simulink model "hpt_1to1_topology"  (R2025a)
settings: Solver=ode23tb  StartTime=0.0  StopTime=0.2  RelTol=1e-3
libraries: spsLinearTransformerLib x9, spsGroundLib x4, spsThreePhaseVIMeasurementLib x3, spsSeriesRLCBranchLib x2, spsThreePhaseSeriesRLCBranchLib x2, spsUniversalBridgeLib x2, spsIGBTLib x1, spsThreePhaseSourceLib x1, spsThreePhaseSeriesRLCLoadLib x1, spsVoltageMeasurementLib x1, spspowerguiLib x1
settings Model: Creator=m1391  LastModifiedBy=m1391

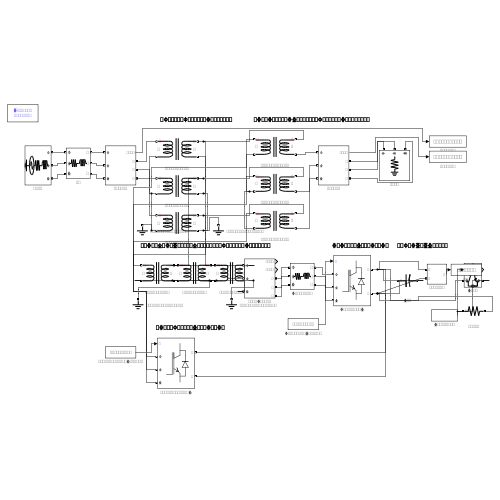
[thumbnail: Simulink's stored preview of the top-level diagram]
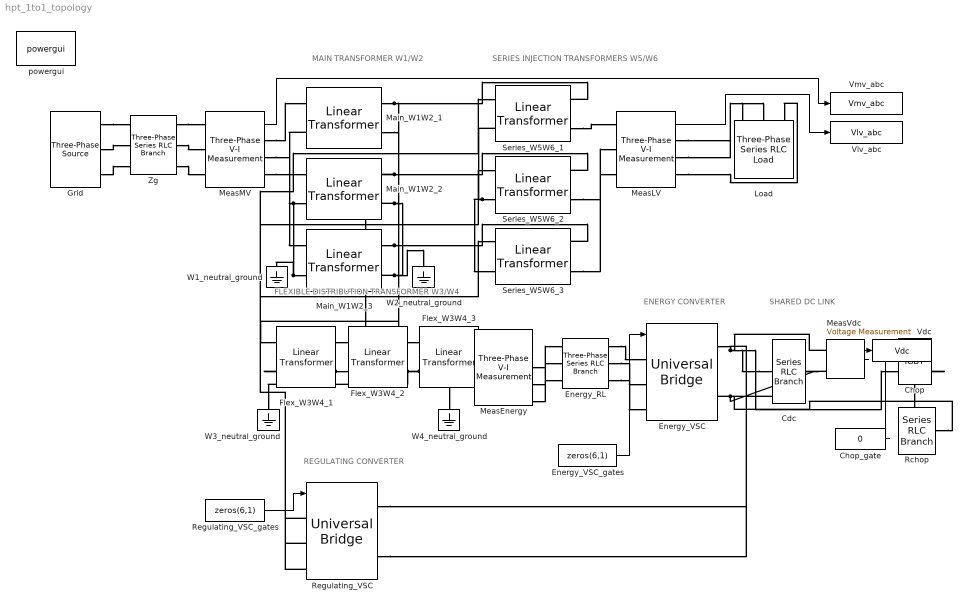
== system hpt_1to1_topology ==
  note: MAIN TRANSFORMER W1/W2
  note: FLEXIBLE DISTRIBUTION TRANSFORMER W3/W4
  note: SERIES INJECTION TRANSFORMERS W5/W6
  note: ENERGY CONVERTER
  note: REGULATING CONVERTER
  note: SHARED DC LINK
  Cdc : spsSeriesRLCBranchLib/Series RLC Branch  LConnTagsString=__new0  RConnTagsString=__new0  BranchType=C  Resistance=1  Inductance=1e-3  SetiL0=off  InitialCurrent=0  Capacitance=0.0022  Setx0=on  InitialVoltage=800  Measurements=None
  Chop : spsIGBTLib/IGBT  Ron=0.001  Lon=0  Vf=1  Tf=1e-6  Tt=2e-6  IC=0  Rs=1e5  Cs=inf  Measurements=on
  Chop_gate : Constant  Value=0
  Energy_RL : spsThreePhaseSeriesRLCBranchLib/Three-Phase Series RLC Branch  LConnTagsString=A|B|C  RConnTagsString=A|B|C  BranchType=RL  Resistance=0.05  Inductance=0.003  Capacitance=1e-6  Measurements=None
  Energy_VSC : spsUniversalBridgeLib/Universal Bridge  Arms=3  SnubberResistance=1e5  SnubberCapacitance=inf  Device=IGBT / Diodes  Ron=1e-3  Lon=0  ForwardVoltages="[  0  0  ]"  ForwardVoltage=0  GTOparameters=[ 10e-6 , 20e-6 ]  IGBTparameters=[ 1e-6 , 2e-6 ]  Measurements=None  Measurements_2=None  converterType=Rectifier
  Energy_VSC_gates : Constant  Value=zeros(6,1)
  Flex_W3W4_1 : spsLinearTransformerLib/Linear Transformer  UNITS=pu  NominalPower=[40000,50]  winding1=[230.9401,0.005,0.02]  winding2=[230.9401,0.005,0.02]  ThreeWindings=off  winding3=[ 315e3 0.002 0.08 ]  RmLm=[ 500 500 ]  Measurements=None  DataType=off
  Flex_W3W4_2 : spsLinearTransformerLib/Linear Transformer  UNITS=pu  NominalPower=[40000,50]  winding1=[230.9401,0.005,0.02]  winding2=[230.9401,0.005,0.02]  ThreeWindings=off  winding3=[ 315e3 0.002 0.08 ]  RmLm=[ 500 500 ]  Measurements=None  DataType=off
  Flex_W3W4_3 : spsLinearTransformerLib/Linear Transformer  UNITS=pu  NominalPower=[40000,50]  winding1=[230.9401,0.005,0.02]  winding2=[230.9401,0.005,0.02]  ThreeWindings=off  winding3=[ 315e3 0.002 0.08 ]  RmLm=[ 500 500 ]  Measurements=None  DataType=off
  Grid : spsThreePhaseSourceLib/Three-Phase Source  InternalConnection=Yg  VoltagePhases=off  Voltage=10000  PhaseAngle=0  Voltage_phases=[25e3 25e3 25e3]/sqrt(3)  PhaseAngles_phases=[0 -120 +120]  Frequency=50  NonIdealSource=on  SpecifyImpedance=off  Resistance=1e-3  Inductance=1e-5  ShortCircuitLevel=100e6  BaseVoltage=25e3  XRratio=7  BusType=swing  Pref=10e3  Qref=0  Prefabc=[10e3, 10e3, 10e3]  Qrefabc=[0, 0, 0]  Qmin=-inf  Qmax=inf
  Load : spsThreePhaseSeriesRLCLoadLib/Three-Phase Series RLC Load  LConnTagsString=A|B|C  Configuration=Y (grounded)  NominalVoltage=400  Vabc=[1e3 1e3 1e3]  Vabcp=[1e3 1e3 1e3]  NominalFrequency=50  UnbalancedPower=off  ActivePower=400000  InductivePower=0  CapacitivePower=0  Pabc=[10e3 9e3 11e3]  QLabc=[100 90 110]  QCabc=[100 90 110]  Pabcp=[10e3 9e3 11e3]  QLabcp=[100 90 110]  QCabcp=[100 90 110]  Measurements=None  LoadType=constant Z
  Main_W1W2_1 : spsLinearTransformerLib/Linear Transformer  UNITS=pu  NominalPower=[133333.3333,50]  winding1=[5773.5027,0.005,0.025]  winding2=[230.9401,0.005,0.025]  ThreeWindings=off  winding3=[ 315e3 0.002 0.08 ]  RmLm=[ 500 500 ]  Measurements=None  DataType=off
  Main_W1W2_2 : spsLinearTransformerLib/Linear Transformer  UNITS=pu  NominalPower=[133333.3333,50]  winding1=[5773.5027,0.005,0.025]  winding2=[230.9401,0.005,0.025]  ThreeWindings=off  winding3=[ 315e3 0.002 0.08 ]  RmLm=[ 500 500 ]  Measurements=None  DataType=off
  Main_W1W2_3 : spsLinearTransformerLib/Linear Transformer  UNITS=pu  NominalPower=[133333.3333,50]  winding1=[5773.5027,0.005,0.025]  winding2=[230.9401,0.005,0.025]  ThreeWindings=off  winding3=[ 315e3 0.002 0.08 ]  RmLm=[ 500 500 ]  Measurements=None  DataType=off
  MeasEnergy : spsThreePhaseVIMeasurementLib/Three-Phase V-I Measurement  VoltageMeasurement=phase-to-ground  SetLabelV=off  LabelV=Vabc  Vpu=off  VpuLL=off  CurrentMeasurement=yes  SetLabelI=off  LabelI=Iabc  Ipu=off  Pbase=100e6  Vbase=500e3  OutputType=Complex  PhasorSimulation=off  PSBequivalent=0
  MeasLV : spsThreePhaseVIMeasurementLib/Three-Phase V-I Measurement  VoltageMeasurement=phase-to-ground  SetLabelV=off  LabelV=Vabc  Vpu=off  VpuLL=off  CurrentMeasurement=no  SetLabelI=off  LabelI=Iabc  Ipu=off  Pbase=100e6  Vbase=500e3  OutputType=Complex  PhasorSimulation=off  PSBequivalent=0
  MeasMV : spsThreePhaseVIMeasurementLib/Three-Phase V-I Measurement  VoltageMeasurement=phase-to-ground  SetLabelV=off  LabelV=Vabc  Vpu=off  VpuLL=off  CurrentMeasurement=no  SetLabelI=off  LabelI=Iabc  Ipu=off  Pbase=100e6  Vbase=500e3  OutputType=Complex  PhasorSimulation=off  PSBequivalent=0
  MeasVdc : spsVoltageMeasurementLib/Voltage Measurement  PhasorSimulation=off  OutputType=Complex  PSBequivalent=0
  Rchop : spsSeriesRLCBranchLib/Series RLC Branch  LConnTagsString=__new0  RConnTagsString=__new0  BranchType=R  Resistance=5.3333  Inductance=1e-3  SetiL0=off  InitialCurrent=0  Capacitance=1e-6  Setx0=off  InitialVoltage=0  Measurements=None
  Regulating_VSC : spsUniversalBridgeLib/Universal Bridge  Arms=3  SnubberResistance=1e5  SnubberCapacitance=inf  Device=IGBT / Diodes  Ron=1e-3  Lon=0  ForwardVoltages="[  0  0  ]"  ForwardVoltage=0  GTOparameters=[ 10e-6 , 20e-6 ]  IGBTparameters=[ 1e-6 , 2e-6 ]  Measurements=None  Measurements_2=None  converterType=Rectifier
  Regulating_VSC_gates : Constant  Value=zeros(6,1)
  Series_W5W6_1 : spsLinearTransformerLib/Linear Transformer  UNITS=pu  NominalPower=[30000,50]  winding1=[400,0.002,0.03]  winding2=[46.2,0.002,0.03]  ThreeWindings=off  winding3=[ 315e3 0.002 0.08 ]  RmLm=[ 500 500 ]  Measurements=None  DataType=off
  Series_W5W6_2 : spsLinearTransformerLib/Linear Transformer  UNITS=pu  NominalPower=[30000,50]  winding1=[400,0.002,0.03]  winding2=[46.2,0.002,0.03]  ThreeWindings=off  winding3=[ 315e3 0.002 0.08 ]  RmLm=[ 500 500 ]  Measurements=None  DataType=off
  Series_W5W6_3 : spsLinearTransformerLib/Linear Transformer  UNITS=pu  NominalPower=[30000,50]  winding1=[400,0.002,0.03]  winding2=[46.2,0.002,0.03]  ThreeWindings=off  winding3=[ 315e3 0.002 0.08 ]  RmLm=[ 500 500 ]  Measurements=None  DataType=off
  Vdc : ToWorkspace  VariableName=Vdc  SampleTime=2e-05
  Vlv_abc : ToWorkspace  VariableName=Vlv_abc  SampleTime=2e-05
  Vmv_abc : ToWorkspace  VariableName=Vmv_abc  SampleTime=2e-05
  W1_neutral_ground : spsGroundLib/Ground  LConnTagsString=a
  W2_neutral_ground : spsGroundLib/Ground  LConnTagsString=a
  W3_neutral_ground : spsGroundLib/Ground  LConnTagsString=a
  W4_neutral_ground : spsGroundLib/Ground  LConnTagsString=a
  Zg : spsThreePhaseSeriesRLCBranchLib/Three-Phase Series RLC Branch  LConnTagsString=A|B|C  RConnTagsString=A|B|C  BranchType=RL  Resistance=11.7851  Inductance=0.26259  Capacitance=1e-6  Measurements=None
  powergui : spspowerguiLib/powergui  Priority=1  SimulationMode=Discrete  SampleTime=2e-05  frequency=60  Iterations=50  frequencyindice=60  Pbase=100e6  ErrMax=1e-4  UnitsV=kV  UnitsW=MW  buscounter=0  FunctionMessages=off  echomessages=off  EnableUseOfTLC=off  CurrentSourceSwitches=off  DisableSnubberDevices=off  DisableRonSwitches=off  DisableVfSwitches=off  DisplayEquations=off  AutomaticDiscreteSolvers=off  SolverType=Tustin/Backward Euler (TBE)  Interpol=off  ExternalGateDelay=off  methode=off  Ts=100  x0status=blocks  SPID=on  SwTol=0  HookPort=off  NonlinearTolerance=1e-4  nMaxIteration=100  ContinueOnMaxIteration=off  RestoreLinks=warning  ResistiveCurrentMeasurement=off  Frange=[0:2:500]  Ylog=off  Xlog=on  ShowGrid=off  save=off  variable=ZData  structure=0  ZoomFFT=off  StartTime=0.0  cycles=1  DisplayStyle=1  fundamental=60  FreqAxis=off  MaxFrequency=1000  frequencyindicesteady=1  RmsSteady=1  display=off
  wires:
  Energy_VSC_gates/1 -> Energy_VSC/1
  Regulating_VSC_gates/1 -> Regulating_VSC/1
  Chop_gate/1 -> Chop/1
  MeasMV/1 -> Vmv_abc/1
  MeasLV/1 -> Vlv_abc/1
  MeasVdc/1 -> Vdc/1
  connections:
  Grid/RConn1 -- Zg/LConn1
  Zg/RConn1 -- MeasMV/LConn1
  MeasMV/RConn1 -- Main_W1W2_1/LConn1
  Series_W5W6_1/RConn1 -- Main_W1W2_1/RConn1 -- Flex_W3W4_1/LConn1
  Series_W5W6_1/RConn2 -- MeasLV/LConn1
  MeasLV/RConn1 -- Load/LConn1
  Flex_W3W4_1/RConn1 -- MeasEnergy/LConn1
  MeasEnergy/RConn1 -- Energy_RL/LConn1
  Energy_RL/RConn1 -- Energy_VSC/LConn1
  Regulating_VSC/LConn1 -- Series_W5W6_1/LConn1
  Grid/RConn2 -- Zg/LConn2
  Zg/RConn2 -- MeasMV/LConn2
  MeasMV/RConn2 -- Main_W1W2_2/LConn1
  Series_W5W6_2/RConn1 -- Main_W1W2_2/RConn1 -- Flex_W3W4_2/LConn1
  Series_W5W6_2/RConn2 -- MeasLV/LConn2
  MeasLV/RConn2 -- Load/LConn2
  Flex_W3W4_2/RConn1 -- MeasEnergy/LConn2
  MeasEnergy/RConn2 -- Energy_RL/LConn2
  Energy_RL/RConn2 -- Energy_VSC/LConn2
  Regulating_VSC/LConn2 -- Series_W5W6_2/LConn1
  Grid/RConn3 -- Zg/LConn3
  Zg/RConn3 -- MeasMV/LConn3
  MeasMV/RConn3 -- Main_W1W2_3/LConn1
  Series_W5W6_3/RConn1 -- Main_W1W2_3/RConn1 -- Flex_W3W4_3/LConn1
  Series_W5W6_3/RConn2 -- MeasLV/LConn3
  MeasLV/RConn3 -- Load/LConn3
  Flex_W3W4_3/RConn1 -- MeasEnergy/LConn3
  MeasEnergy/RConn3 -- Energy_RL/LConn3
  Energy_RL/RConn3 -- Energy_VSC/LConn3
  Regulating_VSC/LConn3 -- Series_W5W6_3/LConn1
  Main_W1W2_2/LConn2 -- Main_W1W2_1/LConn2 -- Main_W1W2_3/LConn2 -- W1_neutral_ground/LConn1
  Main_W1W2_2/RConn2 -- Main_W1W2_1/RConn2 -- Main_W1W2_3/RConn2 -- W2_neutral_ground/LConn1
  Flex_W3W4_2/LConn2 -- Flex_W3W4_1/LConn2 -- Flex_W3W4_3/LConn2 -- W3_neutral_ground/LConn1
  Flex_W3W4_2/RConn2 -- Flex_W3W4_1/RConn2 -- Flex_W3W4_3/RConn2 -- W4_neutral_ground/LConn1
  Series_W5W6_2/LConn2 -- Series_W5W6_1/LConn2 -- Series_W5W6_3/LConn2
  Cdc/LConn1 -- Energy_VSC/RConn1 -- Regulating_VSC/RConn1 -- MeasVdc/LConn1 -- Chop/LConn1
  Cdc/RConn1 -- Regulating_VSC/RConn2 -- MeasVdc/LConn2 -- Energy_VSC/RConn2 -- Rchop/RConn1
  Chop/RConn1 -- Rchop/LConn1
